simulink model "digital_twin_model_v2"  (R2023a)
settings: Solver=FixedStepAuto  StartTime=0.0  StopTime=515  FixedStep=ts  RelTol=1e-3
values from neighbouring files (symbols this model uses):
  Ccell0 = cell0 / v_cell    (= 15384.6153846)    [MainCode.m]
  CG0 = 185    [MainCode.m]
  cg_noGrowth = 10    [MainCode.m]
  CM = 4    [MainCode.m]
  CO0 = .245    (= 0.245)    [MainCode.m]
  count_thresh = 3    [MainCode.m]
  F_fresh_start = 5 * .016 * 60    (= 4.8)    [MainCode.m]
  F_net = F_fresh_start + F_recycle_start    (= 334.8)    [MainCode.m]
  F_recycle_start = 5 * 1.1 * 60    (= 330)    [MainCode.m]
  freshPump_response_increases = 2    [MainCode.m]
  freshPump_response_window = 10    [MainCode.m]
  g_fault_wait_time = 10    [MainCode.m]
  g_flowrate_control_windowsize = 10    [MainCode.m]
  g_lownoise_val = 1.25    [MainCode.m]
  g_numpoints_fail = g_standdev_window_size+1    (= 16)    [MainCode.m]
  g_numpoints_low = 4    [MainCode.m]
  g_prob_arraylen = 15    [MainCode.m]
  g_prob_count = 6    [MainCode.m]
  g_prob_thresh = .45    (= 0.45)    [MainCode.m]
  g_standdev_window_size = 15    [MainCode.m]
  g_standev_tol = 7    [MainCode.m]
  mu_max = 0.0251    [MainCode.m]
  n_size = t_window/ts    (= 2.5)    [MainCode.m]
  n_size_CG = n_size    (= 2.5)    [MainCode.m]
  o2_fail_mean = .008    (= 0.008)    [MainCode.m]
  o2_fault_halfrange = .01    (= 0.01)    [MainCode.m]
  o2_fault_numpoints = 5    [MainCode.m]
  o2_lownoise_val = .0008    (= 0.0008)    [MainCode.m]
  o2_numpoints_low = 6    [MainCode.m]
  o2_prob_arraylen = 10    [MainCode.m]
  o2_prob_count = 6    [MainCode.m]
  o2_prob_thresh = .45    (= 0.45)    [MainCode.m]
  OCR = 2.8e-11    [MainCode.m]
  p_thresh = .4    (= 0.4)    [MainCode.m]
  recPump_drop_val = .02    (= 0.02)    [MainCode.m]
  recPump_rollingavg_samples_buildup = 10    [MainCode.m]
  recPump_smallDrop_size = 0.006    [MainCode.m]
  t_crit_CG = .7    (= 0.7)    [MainCode.m]
  ts = 1    [MainCode.m]
  V = 65.0    (= 65)    [MainCode.m]
  v_cell = 65    [MainCode.m]
  YGC = 155 * 10^-6    (= 0.000155)    [MainCode.m]
undefined symbols (not defined in the file or in its folder): DiscIntNeverNeededParam
libraries: simulink x10, sldrtlib x9, dspstat3 x6, aerolibanimutils x1
(part 2 of 2)

== matlab function digital_twin_model_v2/Attack and Fault Detection System/Glucose Deviation Detection/MATLAB Function ==
  data: dnr input; new_sens_value input; likelihood output; std_dev input; g_prob_arraylen input
function likelihood  = compute_likelihood_rolling(dnr, new_sens_value, std_dev, g_prob_arraylen)

persistent sens_arr;
%fill it if full
if isempty(sens_arr)
    sens_arr = zeros(1, g_prob_arraylen);
end

if (dnr==0)
    %shift array one left and add new element
    shifted_arr = [sens_arr(2:end)];
    sens_arr = [shifted_arr, new_sens_value];

    %compute probability array using values, mean (true value), and stdev
    %.500 is 100%, 0 and 1 are 0%
    p = normcdf(sens_arr, 0, std_dev);
    %shift down to be around 0
    p = p-.5;
    %get net distance away from mean
    p = abs(p);

    %net likelihood is average of array
    likelihood = mean(p);

else
    likelihood=0;

end
end

== matlab function digital_twin_model_v2/Digital Reactor/MATLAB Function2 ==
  data: statement input; num output
function num = tf_num(statement)

if statement==true
    num = 1;
else
    num = 0;
end

== matlab function digital_twin_model_v2/Attack and Fault Detection System/Glucose Abnormally Low Noise Detection/MATLAB Function ==
  data: in input; out output; time input; ignore_over output; aliveTime input
function [out, ignore_over] = ignore15(in, time, aliveTime)

if time>(15+aliveTime)
    out = in;
    ignore_over = 1;
else
    out = 0;
    ignore_over = 0;
end

== matlab function digital_twin_model_v2/Attack and Fault Detection System/Glucose Deviation Detection/MATLAB Function1 ==
  data: dnr input; prob input; isDeviated output; thresh input; thresh_count input
function isDeviated  = fcn(dnr, prob, thresh, thresh_count)

persistent g_count;

if isempty(g_count)
    g_count = 0;
end

if (dnr==0)
    if g_count>=thresh_count
        isDeviated = true;
    else
        isDeviated = false;
        if prob <= thresh
            g_count = 0;
        else %prob > thresh
            g_count = g_count+1;
        end
    end
else
    isDeviated=false;
end

== matlab function digital_twin_model_v2/Attack and Fault Detection System/Glucose Fault Detection/MATLAB Function3 ==
  data: dnr input; isFailed output; stdev_sensor input; stdev_tol input; num_points input
function isFailed = detectGFailure(dnr, stdev_sensor, stdev_tol, num_points)

%create fail count variable
persistent count_g_fail;
%fill it if full
if isempty(count_g_fail)
    count_g_fail = 0;
end

if (dnr==0)
    if count_g_fail==num_points
        isFailed = 1;
    else
        if (stdev_sensor>=stdev_tol)
            count_g_fail = count_g_fail + 1;
        else
            count_g_fail = 0;
        end
        isFailed = 0;
    end
else
    isFailed=0;
end

== matlab function digital_twin_model_v2/Attack and Fault Detection System/Fresh Pump Fault Detection/MATLAB Function ==
  data: dnr input; flowrate_commanded input; freshPumpFail output; glucose_sensor input; samples_to_wait input; samples_increase_in_window input
function freshPumpFail  = noFreshResponse(dnr, flowrate_commanded, glucose_sensor, samples_to_wait, samples_increase_in_window)

%%%%%%% initilizing memory variables
persistent prevFlowrate;
persistent wait_count;
persistent glucoseIncreasesCount;
persistent prevGlucose;
persistent isFailed;

if isempty(prevFlowrate)
    prevFlowrate = flowrate_commanded;
end

if isempty(glucoseIncreasesCount)
    glucoseIncreasesCount = 0;
end

if isempty(prevGlucose)
    prevGlucose = glucose_sensor;
end

if isempty(wait_count)
    wait_count = 0;
end

if isempty(isFailed)
    isFailed = 0;
end

%initialize prevFlowrate
%if prevFlowrate==0
%    prevFlowrate = flowrate_commanded;
%end
%%%%%% end initialization

if(dnr==0)

    if flowrate_commanded>prevFlowrate
        %start the counter
        wait_count = wait_count + 1;
    else
        %if the count hasn't started, and flowrate hasnt increased, keep all 0
        if wait_count==0
            wait_count = 0;
            glucoseIncreasesCount = 0;
            %if the count has started, check for glucose increase
        else
            %increase glucose check counts if it has increased
            if glucose_sensor>prevGlucose
                glucoseIncreasesCount = glucoseIncreasesCount + 1;
            end
            %increase wait counter
            wait_count = wait_count+1;
        end
    end

    %change flowrate increase
    prevFlowrate = flowrate_commanded;
    prevGlucose = glucose_sensor;

    %if we waited all samples and saw enough increases, all good, reset
    if (wait_count>=(samples_to_wait+1) || glucoseIncreasesCount>=samples_increase_in_window)
        %reset all counts
        wait_count = 0;
        glucoseIncreasesCount = 0;
        %if we waited all samples and did not see increases, throw fail flag
    elseif ((wait_count>=samples_to_wait) && (glucoseIncreasesCount<=samples_increase_in_window))
        isFailed = 1;
        glucoseIncreasesCount = samples_increase_in_window + 1;
        wait_count = samples_to_wait + 1;
    end

    if isFailed==1
        wait_count = samples_to_wait + 1;
        glucoseIncreasesCount = samples_increase_in_window + 1;
    end
end

freshPumpFail = isFailed;

%debugging variables

== matlab function digital_twin_model_v2/Attack and Fault Detection System/MATLAB Function2 ==
  data: isFailed input; glucoseFault output; noise_small input; isDeviated input; waitAfterFirst input; glucoseAttacked output; potentialFault output
function [glucoseFault, glucoseAttacked, potentialFault] = glucoseSensorDetection(isFailed, noise_small, isDeviated, waitAfterFirst)

persistent g_fault_wait;
persistent g_fault_sticky;

if isempty(g_fault_wait)
    g_fault_wait = 0;
end

if isempty(g_fault_sticky)
    g_fault_sticky = 0;
end



if (isFailed==0 && noise_small==0 && isDeviated==0)
    glucoseFault = 0;
    glucoseAttacked = 0;
    potentialFault = 0;
else %any are triggered
    g_fault_wait = g_fault_wait + 1;
    glucoseFault = 0;
    glucoseAttacked = 0;
    potentialFault = 1;
end

if (g_fault_wait>=waitAfterFirst)
    potentialFault = 1;
    %first, pure fault detection
    if ((isFailed==1 && noise_small==0 && isDeviated==0) || g_fault_sticky==1)
        glucoseFault = 1;
        glucoseAttacked = 0;
        g_fault_sticky=1;
    else %(isFailed==0 && (noise_small==1 || isDeviated==1))
        glucoseFault = 0;
        glucoseAttacked = 1;
    end
end

== matlab function digital_twin_model_v2/Attack and Fault Detection System/MATLAB Function3 ==
  data: isFailed input; oxygenFault output; noise_small input; isDeviated input; waitAfterFirst input; oxygenAttacked output; potentialFault output
function [oxygenFault, oxygenAttacked, potentialFault] = oxygenSensorDetection(isFailed, noise_small, isDeviated, waitAfterFirst)

persistent o2_fault_wait;

if isempty(o2_fault_wait)
    o2_fault_wait = 0;
end

if (isFailed==0 && noise_small==0 && isDeviated==0)
    oxygenFault = 0;
    oxygenAttacked = 0;
    potentialFault = 0;
else %any are triggered
    o2_fault_wait = o2_fault_wait + 1;
    oxygenFault = 0;
    oxygenAttacked = 0;
    potentialFault = 1;
end

if (o2_fault_wait>=waitAfterFirst)
    potentialFault = 1;
    %first, pure fault detection
    if (isFailed==0 && (noise_small==1 || isDeviated==1))
        oxygenFault = 0;
        oxygenAttacked = 1;
    else %(isFailed==1)
        oxygenFault = 1;
        oxygenAttacked = 0;
    end
end

== matlab function digital_twin_model_v2/Attack and Fault Detection System/Oxygen Abnormally Low Noise Detection1/MATLAB Function ==
  data: in input; out output; time input; ignore_over output; aliveTime input
function [out, ignore_over] = ignore15(in, time, aliveTime)

if time>(15+aliveTime)
    out = in;
    ignore_over = 1;
else
    out = 0;
    ignore_over = 0;
end

== matlab function digital_twin_model_v2/Attack and Fault Detection System/Oxygen Abnormally Low Noise Detection1/MATLAB Function3 ==
  data: dnr input; noiseSmall output; stdev_sensor input; stdev_tol input; num_points input; ignore_over input
function noiseSmall = detectO2Failure(dnr, stdev_sensor, stdev_tol, num_points, ignore_over)

%create fail count variable
persistent count_o2_low;
%fill it if full
if isempty(count_o2_low)
    count_o2_low = 0;
end

if (dnr==0)
    if count_o2_low==num_points
        noiseSmall = 1;
    else
        if (stdev_sensor<=stdev_tol && ignore_over == 1)
            count_o2_low = count_o2_low + 1;
        else
            count_o2_low = 0;
        end
        noiseSmall = 0;
    end
else
    noiseSmall=0;
end

== matlab function digital_twin_model_v2/Attack and Fault Detection System/Oxygen Deviation Detection1/MATLAB Function ==
  data: dnr input; new_sens_value input; likelihood output; std_dev input; o2_prob_arraylen input
function likelihood  = compute_likelihood_rolling(dnr, new_sens_value, std_dev, o2_prob_arraylen)

persistent sens_arr_o2;
%fill it if full
if isempty(sens_arr_o2)
    sens_arr_o2 = zeros(1, o2_prob_arraylen);
end

if (dnr==0)

    %shift array one left and add new element
    shifted_arr = [sens_arr_o2(2:end)];
    sens_arr_o2 = [shifted_arr, new_sens_value];

    %compute probability array using values, mean (true value), and stdev
    %.500 is 100%, 0 and 1 are 0%
    p = normcdf(sens_arr_o2, 0, std_dev);
    %shift down to be around 0
    p = p-.5;
    %get net distance away from mean
    p = abs(p);

    %net likelihood is average of array
    likelihood = mean(p);

else
    likelihood=0;
end
end

== matlab function digital_twin_model_v2/Attack and Fault Detection System/Oxygen Deviation Detection1/MATLAB Function1 ==
  data: dnr input; prob input; isDeviated output; thresh input; thresh_count input
function isDeviated  = fcn(dnr, prob, thresh, thresh_count)

persistent g_count;

if isempty(g_count)
    g_count = 0;
end

if(dnr==0)

    if g_count>=thresh_count
        isDeviated = true;
    else
        isDeviated = false;
        if prob <= thresh
            g_count = 0;
        else %prob > thresh
            g_count = g_count+1;
        end
    end
else
    isDeviated=false;
end

== matlab function digital_twin_model_v2/Attack and Fault Detection System/Oxygen Sensor Failure Detection/MATLAB Function2 ==
  data: dnr input; o2_sensor input; isFailed output; fail_val input; half_range input; num_points input
function isFailed = detectO2Failure(dnr, o2_sensor, fail_val, half_range, num_points)

persistent count_o2_fail;
if isempty(count_o2_fail)
    count_o2_fail = 0;
end

if (dnr==0)
    if count_o2_fail==num_points
        isFailed = 1;
    else
        if (o2_sensor < (fail_val + half_range) && o2_sensor > (fail_val - half_range))
            count_o2_fail = count_o2_fail + 1;
        else
            count_o2_fail = 0;
        end
        isFailed = 0;
    end
else
    isFailed=0;
end

== matlab function digital_twin_model_v2/Attack and Fault Detection System/Recycle Pump Fault Detection/MATLAB Function ==
  data: dnr input; new_flowrate_commanded input; RecyclePumpFail output; oxygen_sensor input; samples_to_wait input; o2_rollavg_drop_spec input; large_drop_val input; largeDrop output
function [RecyclePumpFail, largeDrop]  = noRecycleResponse(dnr, new_flowrate_commanded, oxygen_sensor, samples_to_wait, o2_rollavg_drop_spec, large_drop_val)

%%%%%%% initilizing memory variables
persistent prevFlowrate;
persistent wait_count2;
persistent prevOxygen;
persistent large_drop_occurred;
persistent recyclePumpFailure;
persistent o2_mem;

if isempty(prevFlowrate)
    prevFlowrate = new_flowrate_commanded;
end

if isempty(o2_mem)
    o2_mem = 0;
end

if isempty(recyclePumpFailure)
    recyclePumpFailure = 0;
end

if isempty(large_drop_occurred)
    large_drop_occurred = 0;
end

if isempty(prevOxygen)
    prevOxygen = oxygen_sensor;
end

if isempty(wait_count2)
    wait_count2 = 0;
end

if(dnr==0)
    %if the drop is large enough, triggered the large_drop condition
    %keep large drop toggled if previously toggled
    %if the net flowrate has dropped, it may be attributed to that
    if ((abs(oxygen_sensor - prevOxygen)>large_drop_val || large_drop_occurred==1) && new_flowrate_commanded==prevFlowrate)
        if large_drop_occurred==0 %only remember the last value after the drop
            o2_mem = oxygen_sensor;
        end
        large_drop_occurred = 1;
        %check to see if the oxygen content has dropped to basically zero
        if ((oxygen_sensor<.005) && (oxygen_sensor>-.005))
            recyclePumpFailure=1;
        end
    else
        large_drop_occurred = 0;
    end

    if (large_drop_occurred==1)
        wait_count2 = wait_count2+1;
        if (wait_count2==samples_to_wait)
            if (o2_mem >= (oxygen_sensor+o2_rollavg_drop_spec))
                recyclePumpFailure=1;
            else
                large_drop_occurred=0;
                wait_count2=0;
            end
        end
    end
end
%update previous variables
prevOxygen = oxygen_sensor;
prevFlowrate = new_flowrate_commanded;

%outputs
RecyclePumpFail = recyclePumpFailure;
largeDrop = large_drop_occurred;

== matlab function digital_twin_model_v2/Attack and Fault Detection System/Steady State Detection System1/MATLAB Function2 ==
  data: P_loop_in input; P_loop_out output; ABG input; P output; x input; n input; t_crit input; run_ss_func output
% R. R. Rhinehart, Automated steady and transient state identification in
% noisy processes, in Proceedings of the American Control Conference, 2013,
% no. June 2013, pp. 4477–4493.
%
% Section V

function [P_loop_out, P, run_ss_func]= ssd(P_loop_in, ABG, x, n, t_crit)

if x==0
    P = 0;
    P_loop_out = 0;
    run_ss_func = false;

elseif ABG == 1
    P_loop_out = P_loop_in;
    P = P_loop_in;

    run_ss_func = false;

else
    run_ss_func = true;

    P_array = zeros(length(x),1);

    if n > length(x)
        n = length(x);
    end

    k = 1;
    should_break = 0;
    while 1
        from = k;
        to = from + n - 1;

        if to > length(x)
            to = length(x);
            n = to -from  + 1;
            should_break = 1;
        end

        x_active = x(from:to);

        % By first differencing xt it is possible to unbiasedly1 estimate the slope
        % m of the drift component mt as the arithmetic average of xt − xt−1 with
        % n sampled values of xt in the window which areequally spaced in time
        % i.e., given a uniform sampling period or cycle.
        m = 0;
        for t = 2 : n
            m = m + (x_active(t)-x_active(t-1));
        end
        m = m/n;

        % eq. 3
        mu = (sum(x_active) - sum(1:n)*m)/n;

        % eq. 4
        sd = 0;
        for t = 1 : n
            sd = sd + (x_active(t) - m*t-mu)^2;
        end
        sd = sqrt(sd/(n-2));

        % eq. 5
        y = 0;
        for t = 1 : n
            if abs(x_active(t)-mu) <= t_crit * sd
                y = y + 1;
            end
        end
        y = y/n;

        P_array(from:to,1) = y;

        if should_break == 1
            break;
        end

        k = k + n;
    end
    P = mean(P_array);
    P_loop_out = P;

end

== matlab function digital_twin_model_v2/Attack and Fault Detection System/Glucose Fault Detection/MATLAB Function ==
  data: in input; out output; time input; aliveTime input
function out = ignore15(in, time, aliveTime)

if time>(15 + aliveTime)
    out = in;
else
    out = 0;
end

== matlab function digital_twin_model_v2/Attack and Fault Detection System/Steady State Detection System1/MATLAB Function3 ==
  data: new_count output; SS_prev input; count input; count_thresh input; run_func input; p input; isSteadyState output; p_thresh input
function [new_count, isSteadyState]= fcn(SS_prev,count, count_thresh, run_func, p, p_thresh)



if run_func == true
    if SS_prev == 1 %last state WAS steady
        if p>p_thresh %still SS
            new_count = 0;
        else %changed to notSS
            new_count = count + 1;
        end
    else %last state was notSS
        if p<p_thresh %still notSS
            new_count = 0;
        else %changed to SS
            new_count = count + 1;
        end
    end
    if new_count >= count_thresh
        if SS_prev == 1
            isSteadyState = 0;
        else
            isSteadyState = 1;
        end
    else
        isSteadyState = SS_prev;
    end
else
    new_count = count;
    isSteadyState = SS_prev;
end





















%     if SS_temp_in==0
%         if p<p_thresh
%             isSteadyState = 0;
%             SS_temp_out = 0;
%         else %p > p_thresh
%             isSteadyState = 0;
%             SS_temp_out = 2;
%         end
% 
%     elseif SS_temp_in == 2
%         if p>p_thresh
%             isSteadyState = 1;
%             SS_temp_out = 1;
%         else %p < p_thresh
%             isSteadyState = 0;
%             SS_temp_out = 0;
%         end
%     else %SS_temp_in == 1
%         if p>p_thresh
%             isSteadyState = 1;
%             SS_temp_out = 1;
%         else %p < p_thresh
%             isSteadyState = 1;
%             SS_temp_out = 2;
%         end
%         
%     end
%     
% 
% else
%     isSteadyState = isSteadyState_loop_in;
%     SS_temp_out = SS_temp_in;
% end
% 
% isSteadyState_loop_out = isSteadyState;
% 
% whatLoop_in_was = isSteadyState_loop_in;
% whattempinwas = SS_temp_in;

== matlab function digital_twin_model_v2/Attack and Fault Detection System/Steady State Detection System1/MATLAB Function4 ==
  data: input input; ABG output; n_size input
function ABG = fcn(input, n_size)

if mod(input,n_size)==0
    ABG = -1;
else
    ABG = 1;
end

== matlab function digital_twin_model_v2/Digital Reactor/MATLAB Function3 ==
  data: divide input; out output; mult input
function out = divideNotZero(divide, mult)

if divide==0
    out = 0;
else
    out = mult/divide;
end

== matlab function digital_twin_model_v2/Attack and Fault Detection System/Oxygen Abnormally Low Noise Detection1/MATLAB Function1 ==
  data: DNR input; output output; input input
function output = echoIfDNR(DNR, input)

persistent lastInput1;

if isempty(lastInput1)
    lastInput1=0;
end

if DNR==1
    output = lastInput1;
else %DNR==0
    output = input;
    lastInput1 = input;
end

== matlab function digital_twin_model_v2/Attack and Fault Detection System/Glucose Abnormally Low Noise Detection/MATLAB Function1 ==
  data: DNR input; output output; input input
function output = echoIfDNR(DNR, input)

persistent lastInput2;

if isempty(lastInput2)
    lastInput2=0;
end

if DNR==1
    output = lastInput2;
else %DNR==0
    output = input;
    lastInput2 = input;
end

== matlab function digital_twin_model_v2/Subsystem/MATLAB Function ==
  data: u input; doNotRun output; time input; aliveTime output; aliveTime_mem input
function [doNotRun, aliveTime] = fcn(u, time, aliveTime_mem)

%u is true when time has increased
%u is false when time has NOT started

persistent flag1;

if isempty(flag1)
    flag1=0;
end

if (u==false && flag1==0)
    doNotRun=1;
    aliveTime = time;
else %u==true
    doNotRun=0;
    if (flag1==0)
        aliveTime = time;
    else
        aliveTime = aliveTime_mem;
    end
    flag1 = 1;
end

%flips neg to pos, pos to neg

== matlab function digital_twin_model_v2/recycle initializer/MATLAB Function ==
  data: input input; output output; initial_val input; time input
function output = initializer(input, initial_val, time)

if time<50
    if input==0
        output=initial_val;
    else %input is nonzero
        output = input;
    end
else %time>50
    output = input;
end

== matlab function digital_twin_model_v2/fresh initializer1/MATLAB Function ==
  data: input input; output output; initial_val input; time input
function output = initializer(input, initial_val, time)

if time<50
    if input==0
        output=initial_val;
    else %input is nonzero
        output = input;
    end
else %time>50
    output = input;
end

== matlab function digital_twin_model_v2/recycle or fresh medium1 ==
  data: fresh_flowrate input; recycled_flowrate input; CG0 input; CG_recycled input; CG_inlet output; total_flowrate output
function [CG_inlet, total_flowrate]  = isNewFluid(fresh_flowrate, recycled_flowrate, CG0, CG_recycled)

%net flowrate into reactor is fresh+recycle rates
total_flowrate = fresh_flowrate + recycled_flowrate;

%glucose concentration is sum of each fluid stream's concentrations
CG_inlet = ((fresh_flowrate*CG0) + (recycled_flowrate*CG_recycled)) / total_flowrate;
